simulink model "SwarmSMC2"  (R2022a)
settings: Solver=FixedStepAuto  StartTime=0.0  StopTime=240  FixedStep=0.001  RelTol=1e-3
libraries: slpidlib x41
(part 4 of 4)

== system SwarmSMC2/速度环1 ==
  Vx0 : Inport
  Vy0 : Inport  Port=2
  Vz0 : Inport  Port=3
  Vx : Inport  Port=4
  Vy : Inport  Port=5
  Vz : Inport  Port=6
  fan : Inport  Port=7
  theta : Inport  Port=8
  Constant : Constant  Value=g
  Cos : Trigonometry  Operator=cos
  Cos1 : Trigonometry  Operator=cos
  Divide : Product  Inputs=*/
  Gain1 : Gain  Gain=m
  PID Controller : slpidlib/PID Controller  Controller=PID  Form=Parallel  TimeDomain=Continuous-time  UseExternalTs=off  SampleTime=-1  IntegratorMethod=Forward Euler  FilterMethod=Forward Euler  ControllerParametersSource=internal  P=5  I=0  UseKiTs=off  D=6  N=1581.76882497108  UseFilter=on  TunerSelectOption=Transfer Function Based (PID Tuner App)  InitialConditionSource=internal  InitialConditionForIntegrator=0  InitialConditionForFilter=0  DifferentiatorICPrevScaledInput=0  ExternalReset=none  TrackingMode=off  Kt=1  LimitOutput=off  SatLimitsSource=internal  UpperSaturationLimit=inf  LowerSaturationLimit=-inf  LinearizeAsGain=on  AntiWindupMode=none  Kb=1  POutMin=[]  POutMax=[]  IOutMin=[]  IOutMax=[]  DOutMin=[]  DOutMax=[]  NOutMin=[]  NOutMax=[]  SumOutMin=[]  SumOutMax=[]  SaturationOutMin=[]  SaturationOutMax=[]  PParamMin=[]  PParamMax=[]  IParamMin=[]  IParamMax=[]  DParamMin=[]  DParamMax=[]  NParamMin=[]  NParamMax=[]  KbParamMin=[]  KbParamMax=[]  KtParamMin=[]  KtParamMax=[]  KbOutMin=[]  KbOutMax=[]  KtOutMin=[]  KtOutMax=[]  IntegratorOutMin=[]  IntegratorOutMax=[]  FilterOutMin=[]  FilterOutMax=[]  SumI1OutMin=[]  SumI1OutMax=[]  SumI2OutMin=[]  SumI2OutMax=[]  SumI3OutMin=[]  SumI3OutMax=[]  SumI4OutMin=[]  SumI4OutMax=[]  SumDOutMin=[]  SumDOutMax=[]  DifferentiatorOutMin=[]  DifferentiatorOutMax=[]  FilterDiffOutCoefMin=[]  FilterDiffOutCoefMax=[]  ReciprocalOutMin=[]  ReciprocalOutMax=[]  SumDenOutMin=[]  SumDenOutMax=[]  SumNumOutMin=[]  SumNumOutMax=[]  DivideOutMin=[]  DivideOutMax=[]  UdiffTsProdOutMin=[]  UdiffTsProdOutMax=[]  NTsProdOutMin=[]  NTsProdOutMax=[]  UintegralTsProdOutMin=[]  UintegralTsProdOutMax=[]  UngainTsProdOutMin=[]  UngainTsProdOutMax=[]  IntegratorContinuousStateAttributes=''  IntegratorStateMustResolveToSignalObject=off  IntegratorRTWStateStorageClass=Auto  FilterContinuousStateAttributes=''  FilterStateMustResolveToSignalObject=off  FilterRTWStateStorageClass=Auto  ParallelPVariant=InternalParameters  IdealPVariant=Disabled  IVariant=InternalParameters  DVariant=InternalParameters  IntegratorVariant=Continuous  SatVariant=Disabled  AWVariant=Passthrough  PCopyVariant=Disabled  TRVariant=Disabled  FdbkBlocksVariant=Forward  IdealPFdbkVariant=Disabled  SatFdbkVariant=Disabled  DerivativeFilterVariant=ContFilter  NVariant=InternalParameters  NCopyVariant=Disabled  FilterICVariant=InternalICsFilter  IntegratorICVariant=InternalICs  ExternalResetVariant=Disabled  TRSumVariant=Passthrough  SumFdbkVariant=Disabled  SumVariant=Sum_PID  TsampFilterVariant=InternalTs  TsampNgainVariant=Passthrough  TsampIntegralVariant=Passthrough  ExternalSaturationOutDataTypeStr=Inherit: Same as second input  aMode=0
  PID Controller1 : slpidlib/PID Controller  Controller=PID  Form=Parallel  TimeDomain=Continuous-time  UseExternalTs=off  SampleTime=-1  IntegratorMethod=Forward Euler  FilterMethod=Forward Euler  ControllerParametersSource=internal  P=5  I=0  UseKiTs=off  D=6  N=100  UseFilter=on  TunerSelectOption=Transfer Function Based (PID Tuner App)  InitialConditionSource=internal  InitialConditionForIntegrator=0  InitialConditionForFilter=0  DifferentiatorICPrevScaledInput=0  ExternalReset=none  TrackingMode=off  Kt=1  LimitOutput=off  SatLimitsSource=internal  UpperSaturationLimit=inf  LowerSaturationLimit=-inf  LinearizeAsGain=on  AntiWindupMode=none  Kb=1  POutMin=[]  POutMax=[]  IOutMin=[]  IOutMax=[]  DOutMin=[]  DOutMax=[]  NOutMin=[]  NOutMax=[]  SumOutMin=[]  SumOutMax=[]  SaturationOutMin=[]  SaturationOutMax=[]  PParamMin=[]  PParamMax=[]  IParamMin=[]  IParamMax=[]  DParamMin=[]  DParamMax=[]  NParamMin=[]  NParamMax=[]  KbParamMin=[]  KbParamMax=[]  KtParamMin=[]  KtParamMax=[]  KbOutMin=[]  KbOutMax=[]  KtOutMin=[]  KtOutMax=[]  IntegratorOutMin=[]  IntegratorOutMax=[]  FilterOutMin=[]  FilterOutMax=[]  SumI1OutMin=[]  SumI1OutMax=[]  SumI2OutMin=[]  SumI2OutMax=[]  SumI3OutMin=[]  SumI3OutMax=[]  SumI4OutMin=[]  SumI4OutMax=[]  SumDOutMin=[]  SumDOutMax=[]  DifferentiatorOutMin=[]  DifferentiatorOutMax=[]  FilterDiffOutCoefMin=[]  FilterDiffOutCoefMax=[]  ReciprocalOutMin=[]  ReciprocalOutMax=[]  SumDenOutMin=[]  SumDenOutMax=[]  SumNumOutMin=[]  SumNumOutMax=[]  DivideOutMin=[]  DivideOutMax=[]  UdiffTsProdOutMin=[]  UdiffTsProdOutMax=[]  NTsProdOutMin=[]  NTsProdOutMax=[]  UintegralTsProdOutMin=[]  UintegralTsProdOutMax=[]  UngainTsProdOutMin=[]  UngainTsProdOutMax=[]  IntegratorContinuousStateAttributes=''  IntegratorStateMustResolveToSignalObject=off  IntegratorRTWStateStorageClass=Auto  FilterContinuousStateAttributes=''  FilterStateMustResolveToSignalObject=off  FilterRTWStateStorageClass=Auto  ParallelPVariant=InternalParameters  IdealPVariant=Disabled  IVariant=InternalParameters  DVariant=InternalParameters  IntegratorVariant=Continuous  SatVariant=Disabled  AWVariant=Passthrough  PCopyVariant=Disabled  TRVariant=Disabled  FdbkBlocksVariant=Forward  IdealPFdbkVariant=Disabled  SatFdbkVariant=Disabled  DerivativeFilterVariant=ContFilter  NVariant=InternalParameters  NCopyVariant=Disabled  FilterICVariant=InternalICsFilter  IntegratorICVariant=InternalICs  ExternalResetVariant=Disabled  TRSumVariant=Passthrough  SumFdbkVariant=Disabled  SumVariant=Sum_PID  TsampFilterVariant=InternalTs  TsampNgainVariant=Passthrough  TsampIntegralVariant=Passthrough  ExternalSaturationOutDataTypeStr=Inherit: Same as second input  aMode=0
  PID Controller2 : slpidlib/PID Controller  Controller=PID  Form=Parallel  TimeDomain=Continuous-time  UseExternalTs=off  SampleTime=-1  IntegratorMethod=Forward Euler  FilterMethod=Forward Euler  ControllerParametersSource=internal  P=5  I=1.2  UseKiTs=off  D=4  N=100  UseFilter=on  TunerSelectOption=Transfer Function Based (PID Tuner App)  InitialConditionSource=internal  InitialConditionForIntegrator=0  InitialConditionForFilter=0  DifferentiatorICPrevScaledInput=0  ExternalReset=none  TrackingMode=off  Kt=1  LimitOutput=off  SatLimitsSource=internal  UpperSaturationLimit=inf  LowerSaturationLimit=-inf  LinearizeAsGain=on  AntiWindupMode=none  Kb=1  POutMin=[]  POutMax=[]  IOutMin=[]  IOutMax=[]  DOutMin=[]  DOutMax=[]  NOutMin=[]  NOutMax=[]  SumOutMin=[]  SumOutMax=[]  SaturationOutMin=[]  SaturationOutMax=[]  PParamMin=[]  PParamMax=[]  IParamMin=[]  IParamMax=[]  DParamMin=[]  DParamMax=[]  NParamMin=[]  NParamMax=[]  KbParamMin=[]  KbParamMax=[]  KtParamMin=[]  KtParamMax=[]  KbOutMin=[]  KbOutMax=[]  KtOutMin=[]  KtOutMax=[]  IntegratorOutMin=[]  IntegratorOutMax=[]  FilterOutMin=[]  FilterOutMax=[]  SumI1OutMin=[]  SumI1OutMax=[]  SumI2OutMin=[]  SumI2OutMax=[]  SumI3OutMin=[]  SumI3OutMax=[]  SumI4OutMin=[]  SumI4OutMax=[]  SumDOutMin=[]  SumDOutMax=[]  DifferentiatorOutMin=[]  DifferentiatorOutMax=[]  FilterDiffOutCoefMin=[]  FilterDiffOutCoefMax=[]  ReciprocalOutMin=[]  ReciprocalOutMax=[]  SumDenOutMin=[]  SumDenOutMax=[]  SumNumOutMin=[]  SumNumOutMax=[]  DivideOutMin=[]  DivideOutMax=[]  UdiffTsProdOutMin=[]  UdiffTsProdOutMax=[]  NTsProdOutMin=[]  NTsProdOutMax=[]  UintegralTsProdOutMin=[]  UintegralTsProdOutMax=[]  UngainTsProdOutMin=[]  UngainTsProdOutMax=[]  IntegratorContinuousStateAttributes=''  IntegratorStateMustResolveToSignalObject=off  IntegratorRTWStateStorageClass=Auto  FilterContinuousStateAttributes=''  FilterStateMustResolveToSignalObject=off  FilterRTWStateStorageClass=Auto  ParallelPVariant=InternalParameters  IdealPVariant=Disabled  IVariant=InternalParameters  DVariant=InternalParameters  IntegratorVariant=Continuous  SatVariant=Disabled  AWVariant=Passthrough  PCopyVariant=Disabled  TRVariant=Disabled  FdbkBlocksVariant=Forward  IdealPFdbkVariant=Disabled  SatFdbkVariant=Disabled  DerivativeFilterVariant=ContFilter  NVariant=InternalParameters  NCopyVariant=Disabled  FilterICVariant=InternalICsFilter  IntegratorICVariant=InternalICs  ExternalResetVariant=Disabled  TRSumVariant=Passthrough  SumFdbkVariant=Disabled  SumVariant=Sum_PID  TsampFilterVariant=InternalTs  TsampNgainVariant=Passthrough  TsampIntegralVariant=Passthrough  ExternalSaturationOutDataTypeStr=Inherit: Same as second input  aMode=0
  Product : Product
  Scope : Scope
  Scope1 : Scope
  Sum1 : Sum  Inputs=|+-
  Sum2 : Sum  Inputs=|+-
  Sum3 : Sum  Inputs=|+-
  Sum4 : Sum  Inputs=|++
  ddx : Outport
  ddy : Outport  Port=2
  U1 : Outport  Port=3
  wires:
  PID Controller/1 -> Scope/1, ddx/1
  PID Controller1/1 -> ddy/1
  Vx0/1 -> Sum1/1
  Sum1/1 -> PID Controller/1
  Vx/1 -> Sum1/2
  Vy0/1 -> Sum2/1
  Sum2/1 -> PID Controller1/1
  Vy/1 -> Sum2/2
  Vz0/1 -> Sum3/1
  Sum3/1 -> PID Controller2/1
  Vz/1 -> Sum3/2
  PID Controller2/1 -> Scope1/1, Sum4/1
  Constant/1 -> Sum4/2
  Gain1/1 -> Divide/1
  fan/1 -> Cos/1
  theta/1 -> Cos1/1
  Cos/1 -> Product/1
  Cos1/1 -> Product/2
  Product/1 -> Divide/2
  Divide/1 -> U1/1
  Sum4/1 -> Gain1/1

== system SwarmSMC2/速度环2 ==
  Vx0 : Inport
  Vy0 : Inport  Port=2
  Vz0 : Inport  Port=3
  Vx : Inport  Port=4
  Vy : Inport  Port=5
  Vz : Inport  Port=6
  fan : Inport  Port=7
  theta : Inport  Port=8
  Constant : Constant  Value=g
  Cos : Trigonometry  Operator=cos
  Cos1 : Trigonometry  Operator=cos
  Divide : Product  Inputs=*/
  Gain1 : Gain  Gain=m
  PID Controller : slpidlib/PID Controller  Controller=PID  Form=Parallel  TimeDomain=Continuous-time  UseExternalTs=off  SampleTime=-1  IntegratorMethod=Forward Euler  FilterMethod=Forward Euler  ControllerParametersSource=internal  P=5  I=0  UseKiTs=off  D=6  N=1581.76882497108  UseFilter=on  TunerSelectOption=Transfer Function Based (PID Tuner App)  InitialConditionSource=internal  InitialConditionForIntegrator=0  InitialConditionForFilter=0  DifferentiatorICPrevScaledInput=0  ExternalReset=none  TrackingMode=off  Kt=1  LimitOutput=off  SatLimitsSource=internal  UpperSaturationLimit=inf  LowerSaturationLimit=-inf  LinearizeAsGain=on  AntiWindupMode=none  Kb=1  POutMin=[]  POutMax=[]  IOutMin=[]  IOutMax=[]  DOutMin=[]  DOutMax=[]  NOutMin=[]  NOutMax=[]  SumOutMin=[]  SumOutMax=[]  SaturationOutMin=[]  SaturationOutMax=[]  PParamMin=[]  PParamMax=[]  IParamMin=[]  IParamMax=[]  DParamMin=[]  DParamMax=[]  NParamMin=[]  NParamMax=[]  KbParamMin=[]  KbParamMax=[]  KtParamMin=[]  KtParamMax=[]  KbOutMin=[]  KbOutMax=[]  KtOutMin=[]  KtOutMax=[]  IntegratorOutMin=[]  IntegratorOutMax=[]  FilterOutMin=[]  FilterOutMax=[]  SumI1OutMin=[]  SumI1OutMax=[]  SumI2OutMin=[]  SumI2OutMax=[]  SumI3OutMin=[]  SumI3OutMax=[]  SumI4OutMin=[]  SumI4OutMax=[]  SumDOutMin=[]  SumDOutMax=[]  DifferentiatorOutMin=[]  DifferentiatorOutMax=[]  FilterDiffOutCoefMin=[]  FilterDiffOutCoefMax=[]  ReciprocalOutMin=[]  ReciprocalOutMax=[]  SumDenOutMin=[]  SumDenOutMax=[]  SumNumOutMin=[]  SumNumOutMax=[]  DivideOutMin=[]  DivideOutMax=[]  UdiffTsProdOutMin=[]  UdiffTsProdOutMax=[]  NTsProdOutMin=[]  NTsProdOutMax=[]  UintegralTsProdOutMin=[]  UintegralTsProdOutMax=[]  UngainTsProdOutMin=[]  UngainTsProdOutMax=[]  IntegratorContinuousStateAttributes=''  IntegratorStateMustResolveToSignalObject=off  IntegratorRTWStateStorageClass=Auto  FilterContinuousStateAttributes=''  FilterStateMustResolveToSignalObject=off  FilterRTWStateStorageClass=Auto  ParallelPVariant=InternalParameters  IdealPVariant=Disabled  IVariant=InternalParameters  DVariant=InternalParameters  IntegratorVariant=Continuous  SatVariant=Disabled  AWVariant=Passthrough  PCopyVariant=Disabled  TRVariant=Disabled  FdbkBlocksVariant=Forward  IdealPFdbkVariant=Disabled  SatFdbkVariant=Disabled  DerivativeFilterVariant=ContFilter  NVariant=InternalParameters  NCopyVariant=Disabled  FilterICVariant=InternalICsFilter  IntegratorICVariant=InternalICs  ExternalResetVariant=Disabled  TRSumVariant=Passthrough  SumFdbkVariant=Disabled  SumVariant=Sum_PID  TsampFilterVariant=InternalTs  TsampNgainVariant=Passthrough  TsampIntegralVariant=Passthrough  ExternalSaturationOutDataTypeStr=Inherit: Same as second input  aMode=0
  PID Controller1 : slpidlib/PID Controller  Controller=PID  Form=Parallel  TimeDomain=Continuous-time  UseExternalTs=off  SampleTime=-1  IntegratorMethod=Forward Euler  FilterMethod=Forward Euler  ControllerParametersSource=internal  P=5  I=0  UseKiTs=off  D=6  N=100  UseFilter=on  TunerSelectOption=Transfer Function Based (PID Tuner App)  InitialConditionSource=internal  InitialConditionForIntegrator=0  InitialConditionForFilter=0  DifferentiatorICPrevScaledInput=0  ExternalReset=none  TrackingMode=off  Kt=1  LimitOutput=off  SatLimitsSource=internal  UpperSaturationLimit=inf  LowerSaturationLimit=-inf  LinearizeAsGain=on  AntiWindupMode=none  Kb=1  POutMin=[]  POutMax=[]  IOutMin=[]  IOutMax=[]  DOutMin=[]  DOutMax=[]  NOutMin=[]  NOutMax=[]  SumOutMin=[]  SumOutMax=[]  SaturationOutMin=[]  SaturationOutMax=[]  PParamMin=[]  PParamMax=[]  IParamMin=[]  IParamMax=[]  DParamMin=[]  DParamMax=[]  NParamMin=[]  NParamMax=[]  KbParamMin=[]  KbParamMax=[]  KtParamMin=[]  KtParamMax=[]  KbOutMin=[]  KbOutMax=[]  KtOutMin=[]  KtOutMax=[]  IntegratorOutMin=[]  IntegratorOutMax=[]  FilterOutMin=[]  FilterOutMax=[]  SumI1OutMin=[]  SumI1OutMax=[]  SumI2OutMin=[]  SumI2OutMax=[]  SumI3OutMin=[]  SumI3OutMax=[]  SumI4OutMin=[]  SumI4OutMax=[]  SumDOutMin=[]  SumDOutMax=[]  DifferentiatorOutMin=[]  DifferentiatorOutMax=[]  FilterDiffOutCoefMin=[]  FilterDiffOutCoefMax=[]  ReciprocalOutMin=[]  ReciprocalOutMax=[]  SumDenOutMin=[]  SumDenOutMax=[]  SumNumOutMin=[]  SumNumOutMax=[]  DivideOutMin=[]  DivideOutMax=[]  UdiffTsProdOutMin=[]  UdiffTsProdOutMax=[]  NTsProdOutMin=[]  NTsProdOutMax=[]  UintegralTsProdOutMin=[]  UintegralTsProdOutMax=[]  UngainTsProdOutMin=[]  UngainTsProdOutMax=[]  IntegratorContinuousStateAttributes=''  IntegratorStateMustResolveToSignalObject=off  IntegratorRTWStateStorageClass=Auto  FilterContinuousStateAttributes=''  FilterStateMustResolveToSignalObject=off  FilterRTWStateStorageClass=Auto  ParallelPVariant=InternalParameters  IdealPVariant=Disabled  IVariant=InternalParameters  DVariant=InternalParameters  IntegratorVariant=Continuous  SatVariant=Disabled  AWVariant=Passthrough  PCopyVariant=Disabled  TRVariant=Disabled  FdbkBlocksVariant=Forward  IdealPFdbkVariant=Disabled  SatFdbkVariant=Disabled  DerivativeFilterVariant=ContFilter  NVariant=InternalParameters  NCopyVariant=Disabled  FilterICVariant=InternalICsFilter  IntegratorICVariant=InternalICs  ExternalResetVariant=Disabled  TRSumVariant=Passthrough  SumFdbkVariant=Disabled  SumVariant=Sum_PID  TsampFilterVariant=InternalTs  TsampNgainVariant=Passthrough  TsampIntegralVariant=Passthrough  ExternalSaturationOutDataTypeStr=Inherit: Same as second input  aMode=0
  PID Controller2 : slpidlib/PID Controller  Controller=PID  Form=Parallel  TimeDomain=Continuous-time  UseExternalTs=off  SampleTime=-1  IntegratorMethod=Forward Euler  FilterMethod=Forward Euler  ControllerParametersSource=internal  P=5  I=1.2  UseKiTs=off  D=4  N=100  UseFilter=on  TunerSelectOption=Transfer Function Based (PID Tuner App)  InitialConditionSource=internal  InitialConditionForIntegrator=0  InitialConditionForFilter=0  DifferentiatorICPrevScaledInput=0  ExternalReset=none  TrackingMode=off  Kt=1  LimitOutput=off  SatLimitsSource=internal  UpperSaturationLimit=inf  LowerSaturationLimit=-inf  LinearizeAsGain=on  AntiWindupMode=none  Kb=1  POutMin=[]  POutMax=[]  IOutMin=[]  IOutMax=[]  DOutMin=[]  DOutMax=[]  NOutMin=[]  NOutMax=[]  SumOutMin=[]  SumOutMax=[]  SaturationOutMin=[]  SaturationOutMax=[]  PParamMin=[]  PParamMax=[]  IParamMin=[]  IParamMax=[]  DParamMin=[]  DParamMax=[]  NParamMin=[]  NParamMax=[]  KbParamMin=[]  KbParamMax=[]  KtParamMin=[]  KtParamMax=[]  KbOutMin=[]  KbOutMax=[]  KtOutMin=[]  KtOutMax=[]  IntegratorOutMin=[]  IntegratorOutMax=[]  FilterOutMin=[]  FilterOutMax=[]  SumI1OutMin=[]  SumI1OutMax=[]  SumI2OutMin=[]  SumI2OutMax=[]  SumI3OutMin=[]  SumI3OutMax=[]  SumI4OutMin=[]  SumI4OutMax=[]  SumDOutMin=[]  SumDOutMax=[]  DifferentiatorOutMin=[]  DifferentiatorOutMax=[]  FilterDiffOutCoefMin=[]  FilterDiffOutCoefMax=[]  ReciprocalOutMin=[]  ReciprocalOutMax=[]  SumDenOutMin=[]  SumDenOutMax=[]  SumNumOutMin=[]  SumNumOutMax=[]  DivideOutMin=[]  DivideOutMax=[]  UdiffTsProdOutMin=[]  UdiffTsProdOutMax=[]  NTsProdOutMin=[]  NTsProdOutMax=[]  UintegralTsProdOutMin=[]  UintegralTsProdOutMax=[]  UngainTsProdOutMin=[]  UngainTsProdOutMax=[]  IntegratorContinuousStateAttributes=''  IntegratorStateMustResolveToSignalObject=off  IntegratorRTWStateStorageClass=Auto  FilterContinuousStateAttributes=''  FilterStateMustResolveToSignalObject=off  FilterRTWStateStorageClass=Auto  ParallelPVariant=InternalParameters  IdealPVariant=Disabled  IVariant=InternalParameters  DVariant=InternalParameters  IntegratorVariant=Continuous  SatVariant=Disabled  AWVariant=Passthrough  PCopyVariant=Disabled  TRVariant=Disabled  FdbkBlocksVariant=Forward  IdealPFdbkVariant=Disabled  SatFdbkVariant=Disabled  DerivativeFilterVariant=ContFilter  NVariant=InternalParameters  NCopyVariant=Disabled  FilterICVariant=InternalICsFilter  IntegratorICVariant=InternalICs  ExternalResetVariant=Disabled  TRSumVariant=Passthrough  SumFdbkVariant=Disabled  SumVariant=Sum_PID  TsampFilterVariant=InternalTs  TsampNgainVariant=Passthrough  TsampIntegralVariant=Passthrough  ExternalSaturationOutDataTypeStr=Inherit: Same as second input  aMode=0
  Product : Product
  Scope : Scope
  Scope1 : Scope
  Sum1 : Sum  Inputs=|+-
  Sum2 : Sum  Inputs=|+-
  Sum3 : Sum  Inputs=|+-
  Sum4 : Sum  Inputs=|++
  ddx : Outport
  ddy : Outport  Port=2
  U1 : Outport  Port=3
  wires:
  PID Controller/1 -> Scope/1, ddx/1
  PID Controller1/1 -> ddy/1
  Vx0/1 -> Sum1/1
  Sum1/1 -> PID Controller/1
  Vx/1 -> Sum1/2
  Vy0/1 -> Sum2/1
  Sum2/1 -> PID Controller1/1
  Vy/1 -> Sum2/2
  Vz0/1 -> Sum3/1
  Sum3/1 -> PID Controller2/1
  Vz/1 -> Sum3/2
  PID Controller2/1 -> Scope1/1, Sum4/1
  Constant/1 -> Sum4/2
  Gain1/1 -> Divide/1
  fan/1 -> Cos/1
  theta/1 -> Cos1/1
  Cos/1 -> Product/1
  Cos1/1 -> Product/2
  Product/1 -> Divide/2
  Divide/1 -> U1/1
  Sum4/1 -> Gain1/1

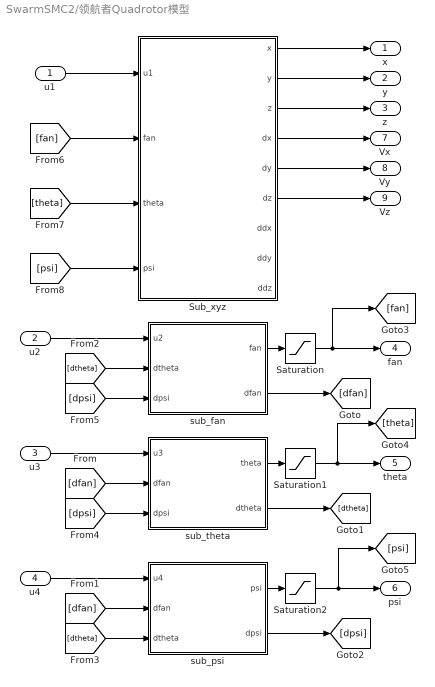
== system SwarmSMC2/领航者Quadrotor模型 ==
  u1 : Inport
  u2 : Inport  Port=2
  u3 : Inport  Port=3
  u4 : Inport  Port=4
  Saturation : Saturate  UpperLimit=inf  LowerLimit=-inf
  Saturation1 : Saturate  UpperLimit=pi/2  LowerLimit=-pi/2
  Saturation2 : Saturate  UpperLimit=pi  LowerLimit=-pi
  Sub_xyz : Subsystem
  sub_fan : Subsystem
  sub_psi : Subsystem
  sub_theta : Subsystem
  x : Outport
  y : Outport  Port=2
  z : Outport  Port=3
  fan : Outport  Port=4
  theta : Outport  Port=5
  psi : Outport  Port=6
  Vx : Outport  Port=7
  Vy : Outport  Port=8
  Vz : Outport  Port=9
  wires:
  u2/1 -> sub_fan/1(u2)
  u3/1 -> sub_theta/1(u3)
  u4/1 -> sub_psi/1(u4)
  sub_fan/1(fan) -> Saturation/1
  sub_theta/1(theta) -> Saturation1/1
  sub_psi/1(psi) -> Saturation2/1
  sub_fan/2(dfan) -> [dfan]
  [dfan] -> sub_theta/2(dfan)
  [dfan] -> sub_psi/2(dfan)
  sub_theta/2(dtheta) -> [dtheta]
  sub_psi/2(dpsi) -> [dpsi]
  [dtheta] -> sub_fan/2(dtheta)
  [dtheta] -> sub_psi/3(dtheta)
  [dpsi] -> sub_theta/3(dpsi)
  [dpsi] -> sub_fan/3(dpsi)
  u1/1 -> Sub_xyz/1(u1)
  Sub_xyz/1(x) -> x/1
  Sub_xyz/2(y) -> y/1
  Sub_xyz/3(z) -> z/1
  [fan] -> Sub_xyz/2(fan)
  [theta] -> Sub_xyz/3(theta)
  [psi] -> Sub_xyz/4(psi)
  Saturation/1 -> [fan], fan/1
  Saturation1/1 -> [theta], theta/1
  Saturation2/1 -> [psi], psi/1
  Sub_xyz/4(dx) -> Vx/1
  Sub_xyz/5(dy) -> Vy/1
  Sub_xyz/6(dz) -> Vz/1

== system SwarmSMC2/领航者Quadrotor模型1 ==
  u1 : Inport
  u2 : Inport  Port=2
  u3 : Inport  Port=3
  u4 : Inport  Port=4
  Saturation : Saturate  UpperLimit=inf  LowerLimit=-inf
  Saturation1 : Saturate  UpperLimit=pi/2  LowerLimit=-pi/2
  Saturation2 : Saturate  UpperLimit=pi  LowerLimit=-pi
  Sub_xyz : Subsystem
  sub_fan : Subsystem
  sub_psi : Subsystem
  sub_theta : Subsystem
  x : Outport
  y : Outport  Port=2
  z : Outport  Port=3
  fan : Outport  Port=4
  theta : Outport  Port=5
  psi : Outport  Port=6
  wires:
  u2/1 -> sub_fan/1(u2)
  u3/1 -> sub_theta/1(u3)
  u4/1 -> sub_psi/1(u4)
  sub_fan/1(fan) -> Saturation/1
  sub_theta/1(theta) -> Saturation1/1
  sub_psi/1(psi) -> Saturation2/1
  sub_fan/2(dfan) -> [dfan]
  [dfan] -> sub_theta/2(dfan)
  [dfan] -> sub_psi/2(dfan)
  sub_theta/2(dtheta) -> [dtheta]
  sub_psi/2(dpsi) -> [dpsi]
  [dtheta] -> sub_fan/2(dtheta)
  [dtheta] -> sub_psi/3(dtheta)
  [dpsi] -> sub_theta/3(dpsi)
  [dpsi] -> sub_fan/3(dpsi)
  u1/1 -> Sub_xyz/1(u1)
  Sub_xyz/1(x) -> x/1
  Sub_xyz/2(y) -> y/1
  Sub_xyz/3(z) -> z/1
  [fan] -> Sub_xyz/2(fan)
  [theta] -> Sub_xyz/3(theta)
  [psi] -> Sub_xyz/4(psi)
  Saturation/1 -> [fan], fan/1
  Saturation1/1 -> [theta], theta/1
  Saturation2/1 -> [psi], psi/1

== system SwarmSMC2/领航者Quadrotor模型2 ==
  u1 : Inport
  u2 : Inport  Port=2
  u3 : Inport  Port=3
  u4 : Inport  Port=4
  Saturation : Saturate  UpperLimit=inf  LowerLimit=-inf
  Saturation1 : Saturate  UpperLimit=pi/2  LowerLimit=-pi/2
  Saturation2 : Saturate  UpperLimit=pi  LowerLimit=-pi
  Sub_xyz : Subsystem
  sub_fan : Subsystem
  sub_psi : Subsystem
  sub_theta : Subsystem
  x : Outport
  y : Outport  Port=2
  z : Outport  Port=3
  fan : Outport  Port=4
  theta : Outport  Port=5
  psi : Outport  Port=6
  Vx : Outport  Port=7
  Vy : Outport  Port=8
  Vz : Outport  Port=9
  wires:
  u2/1 -> sub_fan/1(u2)
  u3/1 -> sub_theta/1(u3)
  u4/1 -> sub_psi/1(u4)
  sub_fan/1(fan) -> Saturation/1
  sub_theta/1(theta) -> Saturation1/1
  sub_psi/1(psi) -> Saturation2/1
  sub_fan/2(dfan) -> [dfan]
  [dfan] -> sub_theta/2(dfan)
  [dfan] -> sub_psi/2(dfan)
  sub_theta/2(dtheta) -> [dtheta]
  sub_psi/2(dpsi) -> [dpsi]
  [dtheta] -> sub_fan/2(dtheta)
  [dtheta] -> sub_psi/3(dtheta)
  [dpsi] -> sub_theta/3(dpsi)
  [dpsi] -> sub_fan/3(dpsi)
  u1/1 -> Sub_xyz/1(u1)
  Sub_xyz/1(x) -> x/1
  Sub_xyz/2(y) -> y/1
  Sub_xyz/3(z) -> z/1
  [fan] -> Sub_xyz/2(fan)
  [theta] -> Sub_xyz/3(theta)
  [psi] -> Sub_xyz/4(psi)
  Saturation/1 -> [fan], fan/1
  Saturation1/1 -> [theta], theta/1
  Saturation2/1 -> [psi], psi/1
  Sub_xyz/4(dx) -> Vx/1
  Sub_xyz/5(dy) -> Vy/1
  Sub_xyz/6(dz) -> Vz/1

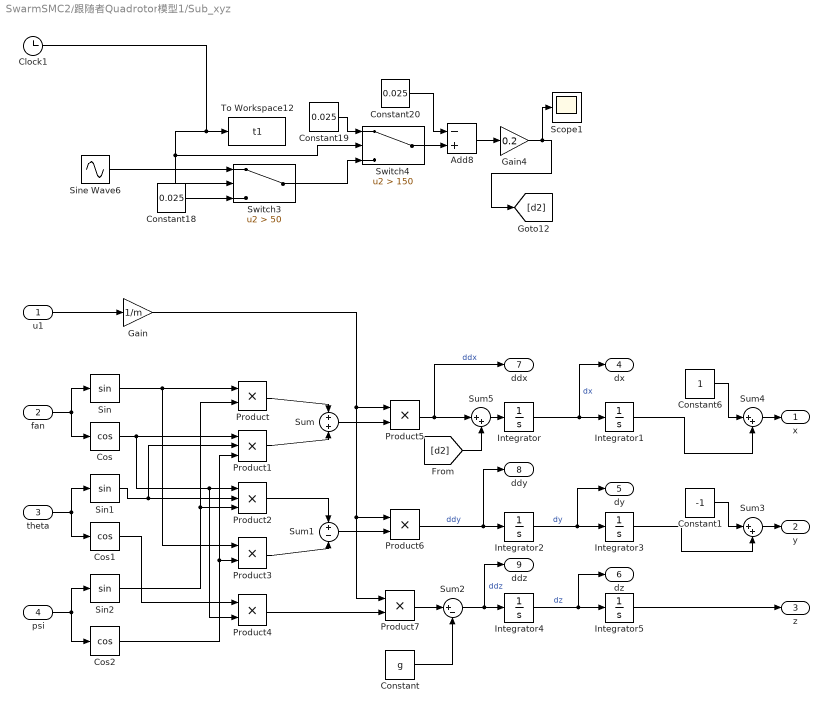
== system SwarmSMC2/跟随者Quadrotor模型1/Sub_xyz ==
  u1 : Inport
  fan : Inport  Port=2
  theta : Inport  Port=3
  psi : Inport  Port=4
  Add8 : Sum  Inputs=-+
  Clock1 : Clock
  Constant : Constant  Value=g
  Constant1 : Constant  Value=-1
  Constant18 : Constant  Value=0.025
  Constant19 : Constant  Value=0.025
  Constant20 : Constant  Value=0.025
  Constant6 : Constant
  Cos : Trigonometry  Operator=cos
  Cos1 : Trigonometry  Operator=cos
  Cos2 : Trigonometry  Operator=cos
  Gain : Gain  Gain=1/m
  Gain4 : Gain  Gain=0.2
  Integrator{,1..5} (6 alike) : Integrator
  Product{,3..7} (6 alike) : Product
  Product1 : Product  Inputs=3
  Product2 : Product  Inputs=3
  Scope1 : Scope
  Sin : Trigonometry
  Sin1 : Trigonometry
  Sin2 : Trigonometry
  Sine Wave6 : Sin  Amplitude=0.5  Frequency=0.5  SampleTime=0
  Sum : Sum  Inputs=+|+
  Sum1 : Sum  Inputs=+|-
  Sum2 : Sum  Inputs=|+-
  Sum3 : Sum  Inputs=|++
  Sum4 : Sum  Inputs=|++
  Sum5 : Sum  Inputs=|++
  Switch3 : Switch  Criteria=u2 > Threshold  Threshold=50  SaturateOnIntegerOverflow=off  InputSameDT=off
  Switch4 : Switch  Criteria=u2 > Threshold  Threshold=150  SaturateOnIntegerOverflow=off  InputSameDT=off
  To Workspace12 : ToWorkspace  VariableName=t1  SampleTime=-1
  x : Outport
  y : Outport  Port=2
  z : Outport  Port=3
  dx : Outport  Port=4
  dy : Outport  Port=5
  dz : Outport  Port=6
  ddx : Outport  Port=7
  ddy : Outport  Port=8
  ddz : Outport  Port=9
  wires:
  u1/1 -> Gain/1
  fan/1 -> Cos/1, Sin/1
  theta/1 -> Cos1/1, Sin1/1
  psi/1 -> Cos2/1, Sin2/1
  Sin/1 -> Product3/1, Product/1
  Sin2/1 -> Product/2, Product2/3
  Cos/1 -> Product4/2, Product2/1, Product1/1
  Sin1/1 -> Product2/2, Product1/2
  Cos2/1 -> Product1/3, Product3/2
  Product/1 -> Sum/1
  Product1/1 -> Sum/2
  Cos1/1 -> Product4/1
  Product2/1 -> Sum1/1
  Product3/1 -> Sum1/2
  Sum/1 -> Product5/2
  Sum1/1 -> Product6/2
  Product4/1 -> Product7/2
  Gain/1 -> Product7/1, Product6/1, Product5/1
  Product5/1 -> Sum5/1, ddx/1  "ddx"
  Integrator/1 -> dx/1, Integrator1/1  "dx"
  Product6/1 -> ddy/1, Integrator2/1  "ddy"
  Integrator2/1 -> dy/1, Integrator3/1  "dy"
  Product7/1 -> Sum2/1
  Constant/1 -> Sum2/2
  Sum2/1 -> ddz/1, Integrator4/1  "ddz"
  Integrator4/1 -> dz/1, Integrator5/1  "dz"
  Integrator3/1 -> Sum3/2
  Integrator1/1 -> Sum4/2
  Integrator5/1 -> z/1
  Constant6/1 -> Sum4/1
  Sum4/1 -> x/1
  Sum3/1 -> y/1
  Constant1/1 -> Sum3/1
  Gain4/1 -> Scope1/1, [d2]
  Add8/1 -> Gain4/1
  Switch3/1 -> Switch4/3
  Constant19/1 -> Switch4/1
  Sine Wave6/1 -> Switch3/1
  Constant18/1 -> Switch3/3
  Switch4/1 -> Add8/2
  Constant20/1 -> Add8/1
  Clock1/1 -> Switch4/2, Switch3/2, To Workspace12/1
  Sum5/1 -> Integrator/1
  [d2] -> Sum5/2

== system SwarmSMC2/跟随者Quadrotor模型1/sub_fan ==
  u2 : Inport
  dtheta : Inport  Port=2
  dpsi : Inport  Port=3
  Gain : Gain  Gain=(Iyy-Izz)/Ixx
  Gain1 : Gain  Gain=1/Ixx
  Integrator : Integrator
  Integrator1 : Integrator
  Product : Product
  Sum : Sum  Inputs=++|
  fan : Outport
  dfan : Outport  Port=2
  wires:
  Sum/1 -> Integrator/1  "ddfan"
  Integrator/1 -> dfan/1, Integrator1/1  "dfan"
  Integrator1/1 -> fan/1  "fan"
  dtheta/1 -> Product/1
  dpsi/1 -> Product/2
  Product/1 -> Gain/1
  Gain/1 -> Sum/2
  u2/1 -> Gain1/1
  Gain1/1 -> Sum/1

== system SwarmSMC2/跟随者Quadrotor模型1/sub_psi ==
  u4 : Inport
  dfan : Inport  Port=2
  dtheta : Inport  Port=3
  Gain : Gain  Gain=(Ixx-Iyy)/Izz
  Gain1 : Gain  Gain=1/Izz
  Integrator : Integrator
  Integrator1 : Integrator
  Product : Product
  Sum : Sum  Inputs=++|
  psi : Outport
  dpsi : Outport  Port=2
  wires:
  Sum/1 -> Integrator/1  "ddpsi"
  Integrator/1 -> dpsi/1, Integrator1/1  "dpsi"
  Integrator1/1 -> psi/1  "psi"
  dfan/1 -> Product/1
  dtheta/1 -> Product/2
  Product/1 -> Gain/1
  Gain/1 -> Sum/2
  u4/1 -> Gain1/1
  Gain1/1 -> Sum/1

== system SwarmSMC2/跟随者Quadrotor模型1/sub_theta ==
  u3 : Inport
  dfan : Inport  Port=2
  dpsi : Inport  Port=3
  Gain : Gain  Gain=(Izz-Ixx)/Iyy
  Gain1 : Gain  Gain=1/Iyy
  Integrator : Integrator
  Integrator1 : Integrator
  Product : Product
  Sum : Sum  Inputs=++|
  theta : Outport
  dtheta : Outport  Port=2
  wires:
  Sum/1 -> Integrator/1  "ddtheta"
  Integrator/1 -> dtheta/1, Integrator1/1  "dtheta"
  Integrator1/1 -> theta/1  "theta"
  dfan/1 -> Product/1
  dpsi/1 -> Product/2
  Product/1 -> Gain/1
  Gain/1 -> Sum/2
  u3/1 -> Gain1/1
  Gain1/1 -> Sum/1

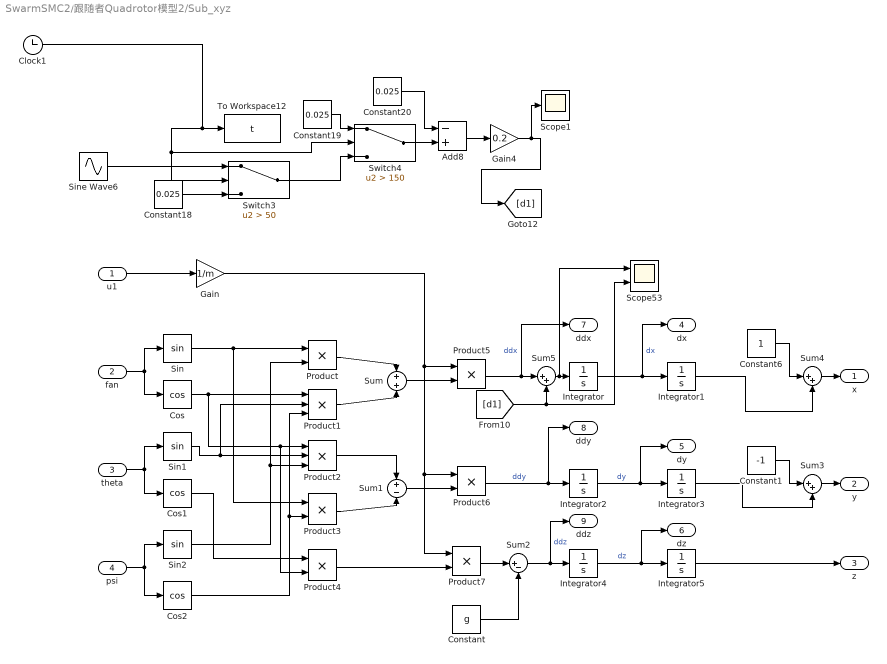
== system SwarmSMC2/跟随者Quadrotor模型2/Sub_xyz ==
  u1 : Inport
  fan : Inport  Port=2
  theta : Inport  Port=3
  psi : Inport  Port=4
  Add8 : Sum  Inputs=-+
  Clock1 : Clock
  Constant : Constant  Value=g
  Constant1 : Constant  Value=-1
  Constant18 : Constant  Value=0.025
  Constant19 : Constant  Value=0.025
  Constant20 : Constant  Value=0.025
  Constant6 : Constant
  Cos : Trigonometry  Operator=cos
  Cos1 : Trigonometry  Operator=cos
  Cos2 : Trigonometry  Operator=cos
  Gain : Gain  Gain=1/m
  Gain4 : Gain  Gain=0.2
  Integrator{,1..5} (6 alike) : Integrator
  Product{,3..7} (6 alike) : Product
  Product1 : Product  Inputs=3
  Product2 : Product  Inputs=3
  Scope1 : Scope
  Scope53 : Scope  NumInputPorts=2
  Sin : Trigonometry
  Sin1 : Trigonometry
  Sin2 : Trigonometry
  Sine Wave6 : Sin  Amplitude=0.5  Frequency=0.5  SampleTime=0
  Sum : Sum  Inputs=+|+
  Sum1 : Sum  Inputs=+|-
  Sum2 : Sum  Inputs=|+-
  Sum3 : Sum  Inputs=|++
  Sum4 : Sum  Inputs=|++
  Sum5 : Sum  Inputs=|++
  Switch3 : Switch  Criteria=u2 > Threshold  Threshold=50  SaturateOnIntegerOverflow=off  InputSameDT=off
  Switch4 : Switch  Criteria=u2 > Threshold  Threshold=150  SaturateOnIntegerOverflow=off  InputSameDT=off
  To Workspace12 : ToWorkspace  VariableName=t  SampleTime=-1
  x : Outport
  y : Outport  Port=2
  z : Outport  Port=3
  dx : Outport  Port=4
  dy : Outport  Port=5
  dz : Outport  Port=6
  ddx : Outport  Port=7
  ddy : Outport  Port=8
  ddz : Outport  Port=9
  wires:
  u1/1 -> Gain/1
  fan/1 -> Cos/1, Sin/1
  theta/1 -> Cos1/1, Sin1/1
  psi/1 -> Cos2/1, Sin2/1
  Sin/1 -> Product3/1, Product/1
  Sin2/1 -> Product/2, Product2/3
  Cos/1 -> Product4/2, Product2/1, Product1/1
  Sin1/1 -> Product2/2, Product1/2
  Cos2/1 -> Product1/3, Product3/2
  Product/1 -> Sum/1
  Product1/1 -> Sum/2
  Cos1/1 -> Product4/1
  Product2/1 -> Sum1/1
  Product3/1 -> Sum1/2
  Sum/1 -> Product5/2
  Sum1/1 -> Product6/2
  Product4/1 -> Product7/2
  Gain/1 -> Product7/1, Product6/1, Product5/1
  Product5/1 -> Sum5/1, ddx/1  "ddx"
  Integrator/1 -> dx/1, Integrator1/1  "dx"
  Product6/1 -> ddy/1, Integrator2/1  "ddy"
  Integrator2/1 -> dy/1, Integrator3/1  "dy"
  Product7/1 -> Sum2/1
  Constant/1 -> Sum2/2
  Sum2/1 -> ddz/1, Integrator4/1  "ddz"
  Integrator4/1 -> dz/1, Integrator5/1  "dz"
  Integrator3/1 -> Sum3/2
  Integrator1/1 -> Sum4/2
  Integrator5/1 -> z/1
  Constant6/1 -> Sum4/1
  Sum4/1 -> x/1
  Sum3/1 -> y/1
  Constant1/1 -> Sum3/1
  [d1] -> Sum5/2, Scope53/2
  Sum5/1 -> Scope53/1, Integrator/1
  Clock1/1 -> Switch4/2, Switch3/2, To Workspace12/1
  Gain4/1 -> Scope1/1, [d1]
  Constant18/1 -> Switch3/3
  Switch4/1 -> Add8/2
  Constant19/1 -> Switch4/1
  Sine Wave6/1 -> Switch3/1
  Switch3/1 -> Switch4/3
  Add8/1 -> Gain4/1
  Constant20/1 -> Add8/1

== system SwarmSMC2/跟随者Quadrotor模型2/sub_fan ==
  u2 : Inport
  dtheta : Inport  Port=2
  dpsi : Inport  Port=3
  Gain : Gain  Gain=(Iyy-Izz)/Ixx
  Gain1 : Gain  Gain=1/Ixx
  Integrator : Integrator
  Integrator1 : Integrator
  Product : Product
  Sum : Sum  Inputs=++|
  fan : Outport
  dfan : Outport  Port=2
  wires:
  Sum/1 -> Integrator/1  "ddfan"
  Integrator/1 -> dfan/1, Integrator1/1  "dfan"
  Integrator1/1 -> fan/1  "fan"
  dtheta/1 -> Product/1
  dpsi/1 -> Product/2
  Product/1 -> Gain/1
  Gain/1 -> Sum/2
  u2/1 -> Gain1/1
  Gain1/1 -> Sum/1

== system SwarmSMC2/跟随者Quadrotor模型2/sub_psi ==
  u4 : Inport
  dfan : Inport  Port=2
  dtheta : Inport  Port=3
  Gain : Gain  Gain=(Ixx-Iyy)/Izz
  Gain1 : Gain  Gain=1/Izz
  Integrator : Integrator
  Integrator1 : Integrator
  Product : Product
  Sum : Sum  Inputs=++|
  psi : Outport
  dpsi : Outport  Port=2
  wires:
  Sum/1 -> Integrator/1  "ddpsi"
  Integrator/1 -> dpsi/1, Integrator1/1  "dpsi"
  Integrator1/1 -> psi/1  "psi"
  dfan/1 -> Product/1
  dtheta/1 -> Product/2
  Product/1 -> Gain/1
  Gain/1 -> Sum/2
  u4/1 -> Gain1/1
  Gain1/1 -> Sum/1

== system SwarmSMC2/跟随者Quadrotor模型2/sub_theta ==
  u3 : Inport
  dfan : Inport  Port=2
  dpsi : Inport  Port=3
  Gain : Gain  Gain=(Izz-Ixx)/Iyy
  Gain1 : Gain  Gain=1/Iyy
  Integrator : Integrator
  Integrator1 : Integrator
  Product : Product
  Sum : Sum  Inputs=++|
  theta : Outport
  dtheta : Outport  Port=2
  wires:
  Sum/1 -> Integrator/1  "ddtheta"
  Integrator/1 -> dtheta/1, Integrator1/1  "dtheta"
  Integrator1/1 -> theta/1  "theta"
  dfan/1 -> Product/1
  dpsi/1 -> Product/2
  Product/1 -> Gain/1
  Gain/1 -> Sum/2
  u3/1 -> Gain1/1
  Gain1/1 -> Sum/1

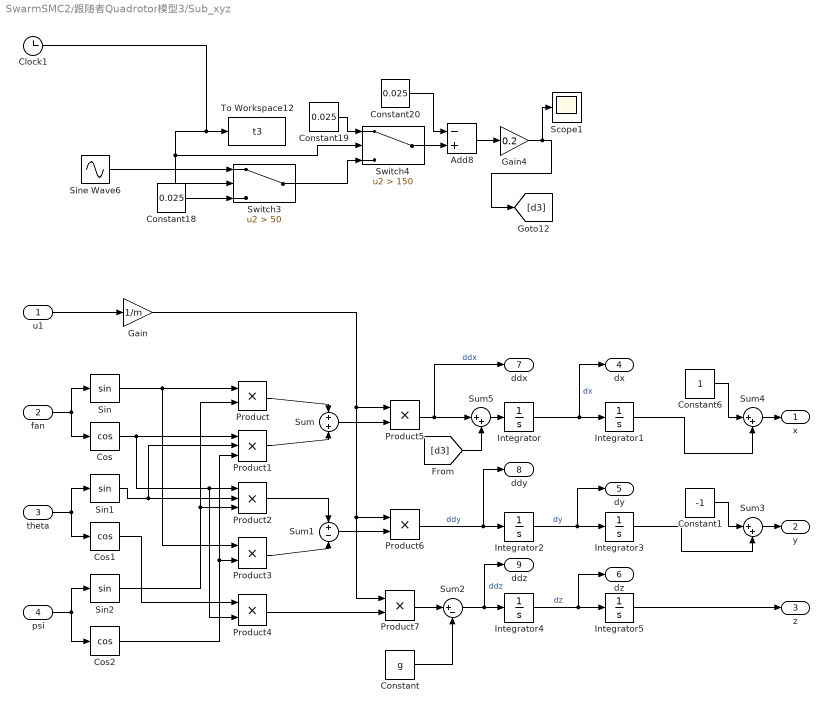
== system SwarmSMC2/跟随者Quadrotor模型3/Sub_xyz ==
  u1 : Inport
  fan : Inport  Port=2
  theta : Inport  Port=3
  psi : Inport  Port=4
  Add8 : Sum  Inputs=-+
  Clock1 : Clock
  Constant : Constant  Value=g
  Constant1 : Constant  Value=-1
  Constant18 : Constant  Value=0.025
  Constant19 : Constant  Value=0.025
  Constant20 : Constant  Value=0.025
  Constant6 : Constant
  Cos : Trigonometry  Operator=cos
  Cos1 : Trigonometry  Operator=cos
  Cos2 : Trigonometry  Operator=cos
  Gain : Gain  Gain=1/m
  Gain4 : Gain  Gain=0.2
  Integrator{,1..5} (6 alike) : Integrator
  Product{,3..7} (6 alike) : Product
  Product1 : Product  Inputs=3
  Product2 : Product  Inputs=3
  Scope1 : Scope
  Sin : Trigonometry
  Sin1 : Trigonometry
  Sin2 : Trigonometry
  Sine Wave6 : Sin  Amplitude=0.5  Frequency=0.5  SampleTime=0
  Sum : Sum  Inputs=+|+
  Sum1 : Sum  Inputs=+|-
  Sum2 : Sum  Inputs=|+-
  Sum3 : Sum  Inputs=|++
  Sum4 : Sum  Inputs=|++
  Sum5 : Sum  Inputs=|++
  Switch3 : Switch  Criteria=u2 > Threshold  Threshold=50  SaturateOnIntegerOverflow=off  InputSameDT=off
  Switch4 : Switch  Criteria=u2 > Threshold  Threshold=150  SaturateOnIntegerOverflow=off  InputSameDT=off
  To Workspace12 : ToWorkspace  VariableName=t3  SampleTime=-1
  x : Outport
  y : Outport  Port=2
  z : Outport  Port=3
  dx : Outport  Port=4
  dy : Outport  Port=5
  dz : Outport  Port=6
  ddx : Outport  Port=7
  ddy : Outport  Port=8
  ddz : Outport  Port=9
  wires:
  u1/1 -> Gain/1
  fan/1 -> Cos/1, Sin/1
  theta/1 -> Cos1/1, Sin1/1
  psi/1 -> Cos2/1, Sin2/1
  Sin/1 -> Product3/1, Product/1
  Sin2/1 -> Product/2, Product2/3
  Cos/1 -> Product4/2, Product2/1, Product1/1
  Sin1/1 -> Product2/2, Product1/2
  Cos2/1 -> Product1/3, Product3/2
  Product/1 -> Sum/1
  Product1/1 -> Sum/2
  Cos1/1 -> Product4/1
  Product2/1 -> Sum1/1
  Product3/1 -> Sum1/2
  Sum/1 -> Product5/2
  Sum1/1 -> Product6/2
  Product4/1 -> Product7/2
  Gain/1 -> Product7/1, Product6/1, Product5/1
  Product5/1 -> Sum5/1, ddx/1  "ddx"
  Integrator/1 -> dx/1, Integrator1/1  "dx"
  Product6/1 -> ddy/1, Integrator2/1  "ddy"
  Integrator2/1 -> dy/1, Integrator3/1  "dy"
  Product7/1 -> Sum2/1
  Constant/1 -> Sum2/2
  Sum2/1 -> ddz/1, Integrator4/1  "ddz"
  Integrator4/1 -> dz/1, Integrator5/1  "dz"
  Integrator3/1 -> Sum3/2
  Integrator1/1 -> Sum4/2
  Integrator5/1 -> z/1
  Constant6/1 -> Sum4/1
  Sum4/1 -> x/1
  Sum3/1 -> y/1
  Constant1/1 -> Sum3/1
  Gain4/1 -> Scope1/1, [d3]
  Add8/1 -> Gain4/1
  Switch3/1 -> Switch4/3
  Constant19/1 -> Switch4/1
  Sine Wave6/1 -> Switch3/1
  Constant18/1 -> Switch3/3
  Switch4/1 -> Add8/2
  Constant20/1 -> Add8/1
  Clock1/1 -> Switch4/2, Switch3/2, To Workspace12/1
  Sum5/1 -> Integrator/1
  [d3] -> Sum5/2

== system SwarmSMC2/跟随者Quadrotor模型3/sub_fan ==
  u2 : Inport
  dtheta : Inport  Port=2
  dpsi : Inport  Port=3
  Gain : Gain  Gain=(Iyy-Izz)/Ixx
  Gain1 : Gain  Gain=1/Ixx
  Integrator : Integrator
  Integrator1 : Integrator
  Product : Product
  Sum : Sum  Inputs=++|
  fan : Outport
  dfan : Outport  Port=2
  wires:
  Sum/1 -> Integrator/1  "ddfan"
  Integrator/1 -> dfan/1, Integrator1/1  "dfan"
  Integrator1/1 -> fan/1  "fan"
  dtheta/1 -> Product/1
  dpsi/1 -> Product/2
  Product/1 -> Gain/1
  Gain/1 -> Sum/2
  u2/1 -> Gain1/1
  Gain1/1 -> Sum/1

== system SwarmSMC2/跟随者Quadrotor模型3/sub_psi ==
  u4 : Inport
  dfan : Inport  Port=2
  dtheta : Inport  Port=3
  Gain : Gain  Gain=(Ixx-Iyy)/Izz
  Gain1 : Gain  Gain=1/Izz
  Integrator : Integrator
  Integrator1 : Integrator
  Product : Product
  Sum : Sum  Inputs=++|
  psi : Outport
  dpsi : Outport  Port=2
  wires:
  Sum/1 -> Integrator/1  "ddpsi"
  Integrator/1 -> dpsi/1, Integrator1/1  "dpsi"
  Integrator1/1 -> psi/1  "psi"
  dfan/1 -> Product/1
  dtheta/1 -> Product/2
  Product/1 -> Gain/1
  Gain/1 -> Sum/2
  u4/1 -> Gain1/1
  Gain1/1 -> Sum/1

== system SwarmSMC2/跟随者Quadrotor模型3/sub_theta ==
  u3 : Inport
  dfan : Inport  Port=2
  dpsi : Inport  Port=3
  Gain : Gain  Gain=(Izz-Ixx)/Iyy
  Gain1 : Gain  Gain=1/Iyy
  Integrator : Integrator
  Integrator1 : Integrator
  Product : Product
  Sum : Sum  Inputs=++|
  theta : Outport
  dtheta : Outport  Port=2
  wires:
  Sum/1 -> Integrator/1  "ddtheta"
  Integrator/1 -> dtheta/1, Integrator1/1  "dtheta"
  Integrator1/1 -> theta/1  "theta"
  dfan/1 -> Product/1
  dpsi/1 -> Product/2
  Product/1 -> Gain/1
  Gain/1 -> Sum/2
  u3/1 -> Gain1/1
  Gain1/1 -> Sum/1

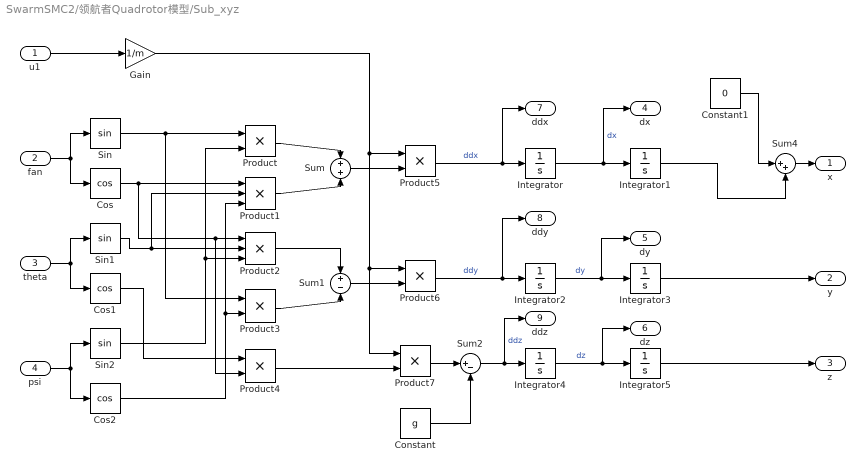
== system SwarmSMC2/领航者Quadrotor模型/Sub_xyz ==
  u1 : Inport
  fan : Inport  Port=2
  theta : Inport  Port=3
  psi : Inport  Port=4
  Constant : Constant  Value=g
  Constant1 : Constant  Value=0
  Cos : Trigonometry  Operator=cos
  Cos1 : Trigonometry  Operator=cos
  Cos2 : Trigonometry  Operator=cos
  Gain : Gain  Gain=1/m
  Integrator{,1..5} (6 alike) : Integrator
  Product{,3..7} (6 alike) : Product
  Product1 : Product  Inputs=3
  Product2 : Product  Inputs=3
  Sin : Trigonometry
  Sin1 : Trigonometry
  Sin2 : Trigonometry
  Sum : Sum  Inputs=+|+
  Sum1 : Sum  Inputs=+|-
  Sum2 : Sum  Inputs=|+-
  Sum4 : Sum  Inputs=|++
  x : Outport
  y : Outport  Port=2
  z : Outport  Port=3
  dx : Outport  Port=4
  dy : Outport  Port=5
  dz : Outport  Port=6
  ddx : Outport  Port=7
  ddy : Outport  Port=8
  ddz : Outport  Port=9
  wires:
  u1/1 -> Gain/1
  fan/1 -> Cos/1, Sin/1
  theta/1 -> Cos1/1, Sin1/1
  psi/1 -> Cos2/1, Sin2/1
  Sin/1 -> Product3/1, Product/1
  Sin2/1 -> Product/2, Product2/3
  Cos/1 -> Product4/2, Product2/1, Product1/1
  Sin1/1 -> Product2/2, Product1/2
  Cos2/1 -> Product1/3, Product3/2
  Product/1 -> Sum/1
  Product1/1 -> Sum/2
  Cos1/1 -> Product4/1
  Product2/1 -> Sum1/1
  Product3/1 -> Sum1/2
  Sum/1 -> Product5/2
  Sum1/1 -> Product6/2
  Product4/1 -> Product7/2
  Gain/1 -> Product7/1, Product6/1, Product5/1
  Product5/1 -> ddx/1, Integrator/1  "ddx"
  Integrator/1 -> dx/1, Integrator1/1  "dx"
  Product6/1 -> ddy/1, Integrator2/1  "ddy"
  Integrator2/1 -> dy/1, Integrator3/1  "dy"
  Product7/1 -> Sum2/1
  Constant/1 -> Sum2/2
  Sum2/1 -> ddz/1, Integrator4/1  "ddz"
  Integrator4/1 -> dz/1, Integrator5/1  "dz"
  Integrator3/1 -> y/1
  Integrator1/1 -> Sum4/2
  Integrator5/1 -> z/1
  Constant1/1 -> Sum4/1
  Sum4/1 -> x/1

== system SwarmSMC2/领航者Quadrotor模型/sub_fan ==
  u2 : Inport
  dtheta : Inport  Port=2
  dpsi : Inport  Port=3
  Gain : Gain  Gain=(Iyy-Izz)/Ixx
  Gain1 : Gain  Gain=1/Ixx
  Integrator : Integrator
  Integrator1 : Integrator
  Product : Product
  Sum : Sum  Inputs=++|
  fan : Outport
  dfan : Outport  Port=2
  wires:
  Sum/1 -> Integrator/1  "ddfan"
  Integrator/1 -> dfan/1, Integrator1/1  "dfan"
  Integrator1/1 -> fan/1  "fan"
  dtheta/1 -> Product/1
  dpsi/1 -> Product/2
  Product/1 -> Gain/1
  Gain/1 -> Sum/2
  u2/1 -> Gain1/1
  Gain1/1 -> Sum/1

== system SwarmSMC2/领航者Quadrotor模型/sub_psi ==
  u4 : Inport
  dfan : Inport  Port=2
  dtheta : Inport  Port=3
  Gain : Gain  Gain=(Ixx-Iyy)/Izz
  Gain1 : Gain  Gain=1/Izz
  Integrator : Integrator
  Integrator1 : Integrator
  Product : Product
  Sum : Sum  Inputs=++|
  psi : Outport
  dpsi : Outport  Port=2
  wires:
  Sum/1 -> Integrator/1  "ddpsi"
  Integrator/1 -> dpsi/1, Integrator1/1  "dpsi"
  Integrator1/1 -> psi/1  "psi"
  dfan/1 -> Product/1
  dtheta/1 -> Product/2
  Product/1 -> Gain/1
  Gain/1 -> Sum/2
  u4/1 -> Gain1/1
  Gain1/1 -> Sum/1

== system SwarmSMC2/领航者Quadrotor模型/sub_theta ==
  u3 : Inport
  dfan : Inport  Port=2
  dpsi : Inport  Port=3
  Gain : Gain  Gain=(Izz-Ixx)/Iyy
  Gain1 : Gain  Gain=1/Iyy
  Integrator : Integrator
  Integrator1 : Integrator
  Product : Product
  Sum : Sum  Inputs=++|
  theta : Outport
  dtheta : Outport  Port=2
  wires:
  Sum/1 -> Integrator/1  "ddtheta"
  Integrator/1 -> dtheta/1, Integrator1/1  "dtheta"
  Integrator1/1 -> theta/1  "theta"
  dfan/1 -> Product/1
  dpsi/1 -> Product/2
  Product/1 -> Gain/1
  Gain/1 -> Sum/2
  u3/1 -> Gain1/1
  Gain1/1 -> Sum/1

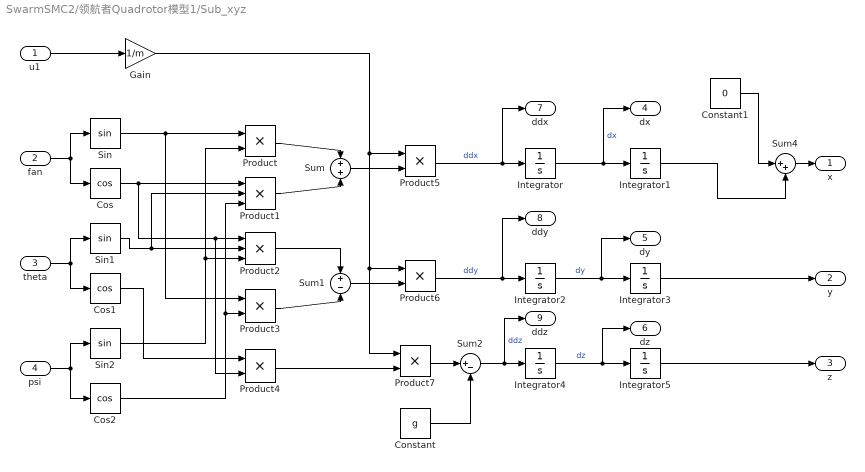
== system SwarmSMC2/领航者Quadrotor模型1/Sub_xyz ==
  u1 : Inport
  fan : Inport  Port=2
  theta : Inport  Port=3
  psi : Inport  Port=4
  Constant : Constant  Value=g
  Constant1 : Constant  Value=0
  Cos : Trigonometry  Operator=cos
  Cos1 : Trigonometry  Operator=cos
  Cos2 : Trigonometry  Operator=cos
  Gain : Gain  Gain=1/m
  Integrator{,1..5} (6 alike) : Integrator
  Product{,3..7} (6 alike) : Product
  Product1 : Product  Inputs=3
  Product2 : Product  Inputs=3
  Sin : Trigonometry
  Sin1 : Trigonometry
  Sin2 : Trigonometry
  Sum : Sum  Inputs=+|+
  Sum1 : Sum  Inputs=+|-
  Sum2 : Sum  Inputs=|+-
  Sum4 : Sum  Inputs=|++
  x : Outport
  y : Outport  Port=2
  z : Outport  Port=3
  dx : Outport  Port=4
  dy : Outport  Port=5
  dz : Outport  Port=6
  ddx : Outport  Port=7
  ddy : Outport  Port=8
  ddz : Outport  Port=9
  wires:
  u1/1 -> Gain/1
  fan/1 -> Cos/1, Sin/1
  theta/1 -> Cos1/1, Sin1/1
  psi/1 -> Cos2/1, Sin2/1
  Sin/1 -> Product3/1, Product/1
  Sin2/1 -> Product/2, Product2/3
  Cos/1 -> Product4/2, Product2/1, Product1/1
  Sin1/1 -> Product2/2, Product1/2
  Cos2/1 -> Product1/3, Product3/2
  Product/1 -> Sum/1
  Product1/1 -> Sum/2
  Cos1/1 -> Product4/1
  Product2/1 -> Sum1/1
  Product3/1 -> Sum1/2
  Sum/1 -> Product5/2
  Sum1/1 -> Product6/2
  Product4/1 -> Product7/2
  Gain/1 -> Product7/1, Product6/1, Product5/1
  Product5/1 -> ddx/1, Integrator/1  "ddx"
  Integrator/1 -> dx/1, Integrator1/1  "dx"
  Product6/1 -> ddy/1, Integrator2/1  "ddy"
  Integrator2/1 -> dy/1, Integrator3/1  "dy"
  Product7/1 -> Sum2/1
  Constant/1 -> Sum2/2
  Sum2/1 -> ddz/1, Integrator4/1  "ddz"
  Integrator4/1 -> dz/1, Integrator5/1  "dz"
  Integrator3/1 -> y/1
  Integrator1/1 -> Sum4/2
  Integrator5/1 -> z/1
  Constant1/1 -> Sum4/1
  Sum4/1 -> x/1

== system SwarmSMC2/领航者Quadrotor模型1/sub_fan ==
  u2 : Inport
  dtheta : Inport  Port=2
  dpsi : Inport  Port=3
  Gain : Gain  Gain=(Iyy-Izz)/Ixx
  Gain1 : Gain  Gain=1/Ixx
  Integrator : Integrator
  Integrator1 : Integrator
  Product : Product
  Sum : Sum  Inputs=++|
  fan : Outport
  dfan : Outport  Port=2
  wires:
  Sum/1 -> Integrator/1  "ddfan"
  Integrator/1 -> dfan/1, Integrator1/1  "dfan"
  Integrator1/1 -> fan/1  "fan"
  dtheta/1 -> Product/1
  dpsi/1 -> Product/2
  Product/1 -> Gain/1
  Gain/1 -> Sum/2
  u2/1 -> Gain1/1
  Gain1/1 -> Sum/1

== system SwarmSMC2/领航者Quadrotor模型1/sub_psi ==
  u4 : Inport
  dfan : Inport  Port=2
  dtheta : Inport  Port=3
  Gain : Gain  Gain=(Ixx-Iyy)/Izz
  Gain1 : Gain  Gain=1/Izz
  Integrator : Integrator
  Integrator1 : Integrator
  Product : Product
  Sum : Sum  Inputs=++|
  psi : Outport
  dpsi : Outport  Port=2
  wires:
  Sum/1 -> Integrator/1  "ddpsi"
  Integrator/1 -> dpsi/1, Integrator1/1  "dpsi"
  Integrator1/1 -> psi/1  "psi"
  dfan/1 -> Product/1
  dtheta/1 -> Product/2
  Product/1 -> Gain/1
  Gain/1 -> Sum/2
  u4/1 -> Gain1/1
  Gain1/1 -> Sum/1

== system SwarmSMC2/领航者Quadrotor模型1/sub_theta ==
  u3 : Inport
  dfan : Inport  Port=2
  dpsi : Inport  Port=3
  Gain : Gain  Gain=(Izz-Ixx)/Iyy
  Gain1 : Gain  Gain=1/Iyy
  Integrator : Integrator
  Integrator1 : Integrator
  Product : Product
  Sum : Sum  Inputs=++|
  theta : Outport
  dtheta : Outport  Port=2
  wires:
  Sum/1 -> Integrator/1  "ddtheta"
  Integrator/1 -> dtheta/1, Integrator1/1  "dtheta"
  Integrator1/1 -> theta/1  "theta"
  dfan/1 -> Product/1
  dpsi/1 -> Product/2
  Product/1 -> Gain/1
  Gain/1 -> Sum/2
  u3/1 -> Gain1/1
  Gain1/1 -> Sum/1

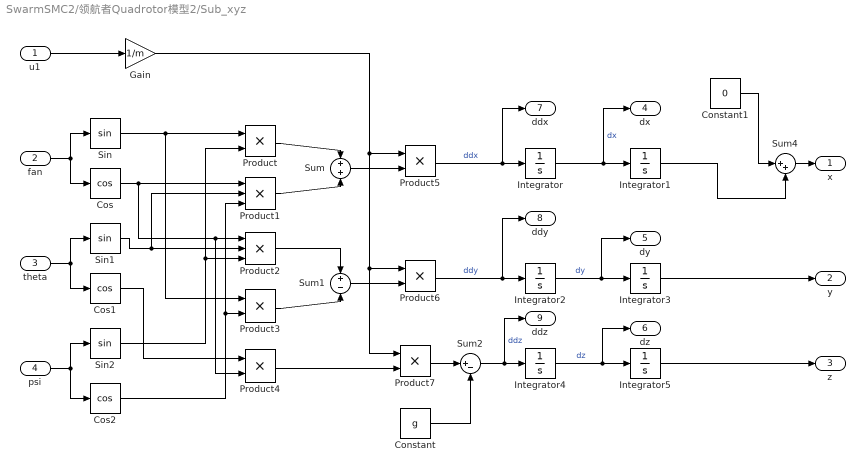
== system SwarmSMC2/领航者Quadrotor模型2/Sub_xyz ==
  u1 : Inport
  fan : Inport  Port=2
  theta : Inport  Port=3
  psi : Inport  Port=4
  Constant : Constant  Value=g
  Constant1 : Constant  Value=0
  Cos : Trigonometry  Operator=cos
  Cos1 : Trigonometry  Operator=cos
  Cos2 : Trigonometry  Operator=cos
  Gain : Gain  Gain=1/m
  Integrator{,1..5} (6 alike) : Integrator
  Product{,3..7} (6 alike) : Product
  Product1 : Product  Inputs=3
  Product2 : Product  Inputs=3
  Sin : Trigonometry
  Sin1 : Trigonometry
  Sin2 : Trigonometry
  Sum : Sum  Inputs=+|+
  Sum1 : Sum  Inputs=+|-
  Sum2 : Sum  Inputs=|+-
  Sum4 : Sum  Inputs=|++
  x : Outport
  y : Outport  Port=2
  z : Outport  Port=3
  dx : Outport  Port=4
  dy : Outport  Port=5
  dz : Outport  Port=6
  ddx : Outport  Port=7
  ddy : Outport  Port=8
  ddz : Outport  Port=9
  wires:
  u1/1 -> Gain/1
  fan/1 -> Cos/1, Sin/1
  theta/1 -> Cos1/1, Sin1/1
  psi/1 -> Cos2/1, Sin2/1
  Sin/1 -> Product3/1, Product/1
  Sin2/1 -> Product/2, Product2/3
  Cos/1 -> Product4/2, Product2/1, Product1/1
  Sin1/1 -> Product2/2, Product1/2
  Cos2/1 -> Product1/3, Product3/2
  Product/1 -> Sum/1
  Product1/1 -> Sum/2
  Cos1/1 -> Product4/1
  Product2/1 -> Sum1/1
  Product3/1 -> Sum1/2
  Sum/1 -> Product5/2
  Sum1/1 -> Product6/2
  Product4/1 -> Product7/2
  Gain/1 -> Product7/1, Product6/1, Product5/1
  Product5/1 -> ddx/1, Integrator/1  "ddx"
  Integrator/1 -> dx/1, Integrator1/1  "dx"
  Product6/1 -> ddy/1, Integrator2/1  "ddy"
  Integrator2/1 -> dy/1, Integrator3/1  "dy"
  Product7/1 -> Sum2/1
  Constant/1 -> Sum2/2
  Sum2/1 -> ddz/1, Integrator4/1  "ddz"
  Integrator4/1 -> dz/1, Integrator5/1  "dz"
  Integrator3/1 -> y/1
  Integrator1/1 -> Sum4/2
  Integrator5/1 -> z/1
  Constant1/1 -> Sum4/1
  Sum4/1 -> x/1

== system SwarmSMC2/领航者Quadrotor模型2/sub_fan ==
  u2 : Inport
  dtheta : Inport  Port=2
  dpsi : Inport  Port=3
  Gain : Gain  Gain=(Iyy-Izz)/Ixx
  Gain1 : Gain  Gain=1/Ixx
  Integrator : Integrator
  Integrator1 : Integrator
  Product : Product
  Sum : Sum  Inputs=++|
  fan : Outport
  dfan : Outport  Port=2
  wires:
  Sum/1 -> Integrator/1  "ddfan"
  Integrator/1 -> dfan/1, Integrator1/1  "dfan"
  Integrator1/1 -> fan/1  "fan"
  dtheta/1 -> Product/1
  dpsi/1 -> Product/2
  Product/1 -> Gain/1
  Gain/1 -> Sum/2
  u2/1 -> Gain1/1
  Gain1/1 -> Sum/1

== system SwarmSMC2/领航者Quadrotor模型2/sub_psi ==
  u4 : Inport
  dfan : Inport  Port=2
  dtheta : Inport  Port=3
  Gain : Gain  Gain=(Ixx-Iyy)/Izz
  Gain1 : Gain  Gain=1/Izz
  Integrator : Integrator
  Integrator1 : Integrator
  Product : Product
  Sum : Sum  Inputs=++|
  psi : Outport
  dpsi : Outport  Port=2
  wires:
  Sum/1 -> Integrator/1  "ddpsi"
  Integrator/1 -> dpsi/1, Integrator1/1  "dpsi"
  Integrator1/1 -> psi/1  "psi"
  dfan/1 -> Product/1
  dtheta/1 -> Product/2
  Product/1 -> Gain/1
  Gain/1 -> Sum/2
  u4/1 -> Gain1/1
  Gain1/1 -> Sum/1

== system SwarmSMC2/领航者Quadrotor模型2/sub_theta ==
  u3 : Inport
  dfan : Inport  Port=2
  dpsi : Inport  Port=3
  Gain : Gain  Gain=(Izz-Ixx)/Iyy
  Gain1 : Gain  Gain=1/Iyy
  Integrator : Integrator
  Integrator1 : Integrator
  Product : Product
  Sum : Sum  Inputs=++|
  theta : Outport
  dtheta : Outport  Port=2
  wires:
  Sum/1 -> Integrator/1  "ddtheta"
  Integrator/1 -> dtheta/1, Integrator1/1  "dtheta"
  Integrator1/1 -> theta/1  "theta"
  dfan/1 -> Product/1
  dpsi/1 -> Product/2
  Product/1 -> Gain/1
  Gain/1 -> Sum/2
  u3/1 -> Gain1/1
  Gain1/1 -> Sum/1

== matlab function SwarmSMC2/编队协同控制器/MATLAB Function2 ==
  data: yd input; uy output; dyd input; ddyd input; y input; dy input
function uy = fcn(yd, dyd, ddyd, y, dy)
ey = y - yd;
dey = dy - dyd;
c =1;
k=0.2;
sy = c*ey + dey;
%滑模
uy = ddyd-c*dey-k*sign(sy);
%反演
% z1 = x - xd;
% dz1 = dx - dxd;
% alpha = dxd - 0.5*z1;
% dalpha = ddxd - 0.5*dz1;
% z2 = dx - alpha;
% ux = m*(dalpha-z1-0.5*z2);

== matlab function SwarmSMC2/编队协同控制器/MATLAB Function1 ==
  data: xd input; ux output; dxd input; ddxd input; x input; dx input; m parameter
function ux = fcn(xd, dxd, ddxd, x, dx, m)
ex = x - xd;
dex = dx - dxd;
c=1;
k=0.2;
sx = c*ex + dex;
%滑模
ux = ddxd-c*dex-k*sign(sx);
%反演
% z1 = x - xd;
% dz1 = dx - dxd;
% alpha = dxd - 0.5*z1;
% dalpha = ddxd - 0.5*dz1;
% z2 = dx - alpha;
% ux = m*(dalpha-z1-0.5*z2);
